simulink model "p8"  (R2020a)
settings: Solver=VariableStepAuto  StartTime=0.0  StopTime=5  RelTol=1e-3
undefined symbols (not defined in the file): Ac, Bc, K, m, n, T, x0
settings Model: Creator=Tomo  LastModifiedBy=Tomo

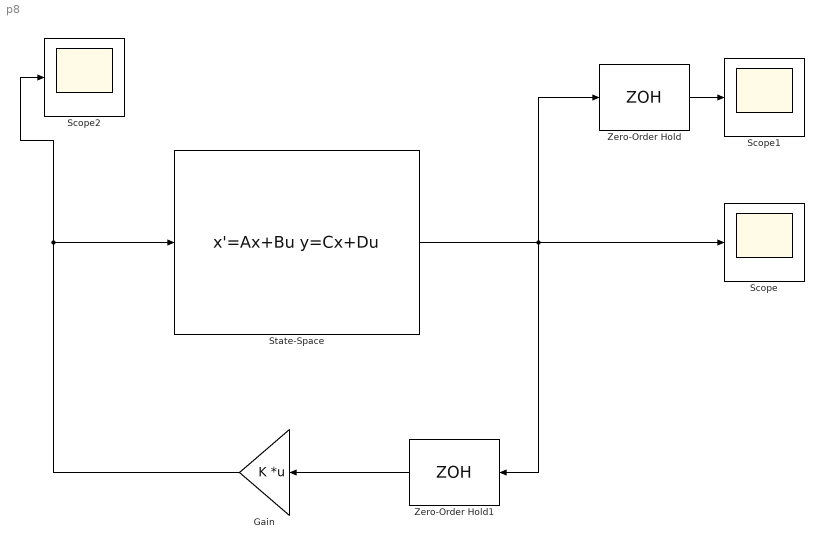
== system p8 ==
  Gain : Gain  Gain=K  Multiplication=Matrix(K*u)
  Scope : Scope
  Scope1 : Scope
  Scope2 : Scope
  State-Space : StateSpace  A=Ac  B=Bc  C=eye(n)  D=zeros(n,m)  InitialCondition=x0
  Zero-Order Hold : ZeroOrderHold  SampleTime=T
  Zero-Order Hold1 : ZeroOrderHold  SampleTime=T
  wires:
  State-Space/1 -> Zero-Order Hold/1, Zero-Order Hold1/1, Scope/1
  Zero-Order Hold1/1 -> Gain/1
  Gain/1 -> Scope2/1, State-Space/1
  Zero-Order Hold/1 -> Scope1/1
